simulink model "dcmotorsimexp"  (Simulink 5.0)
settings: Solver=ode45  SolverMode=SingleTasking  StartTime=0.0  StopTime=Tstop  RelTol=1e-3
values from neighbouring files (symbols this model uses):
  A = [-.0151 -60.5651 0 -32.174 ... (first row only)    [afti16.m]    (also in bmdp02.m = [0.7326   -0.0861; example4.m = [1 -1 0; regulator.m = [0 0; sphericle.m = [0 0 1 0;0 0 0 1 ;-66.2175 66.2175 -0.15 0 ;0 0 0 0])
  B = [-2.516 -13.136 ... (first row only)    [afti16.m]    (also in bmdp02.m = [0.0609;0.0064]; example4.m = [-1 1; regulator.m = [1;0]; sphericle.m = [0 0 0 1]')
  C = [0 1 0 0 ... (first row only)    [afti16.m]    (also in bmdp02.m = lincon(model,'reg',cost,interval,limits); example4.m = lincon(model,'reg',cost,interval,limits); mimo.m = lincon(model,'track',cost,interval,limits); regsiso.m = model.C)
  Cmotorexp = expcon(Cmotor,range,options)    [dcmotor.m]
  D = [0 0 ... (first row only)    [afti16.m]    (also in bmdp02.m = zeros(size(B)); example4.m = zeros(2,2); regulator.m = 0; sphericle.m = 0)
  Vmax = tauam*pi*dshaft^3/16    (= 78.5398163397)    [dcmotor.m]
  Vmin = -Vmax    (= -78.5398163397)    [dcmotor.m]
  x0 = zeros(4,1)    [afti16.m]    (also in bmdp02.m = [1 1]'; dcmotor.m; doubleint.m = [10,-.3]'; doubleintexp.m = [10,-.3]')
libraries: hyblib x1
settings Model: LastModifiedBy=Alberto Bemporad  ExtModeTrigMode=oneshot  ExtModeArmWhenConnect=off  LimitDataPoints=off  IntegerOverflowMsg=none  BooleanDataType=off

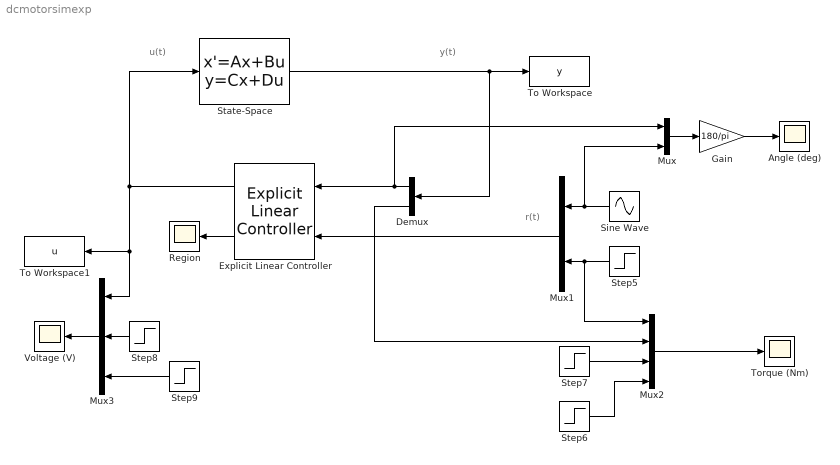
== system dcmotorsimexp ==
  note: u(t)
  note: y(t)
  note: r(t)
  Angle (deg) : Scope
      settings: TimeRange=20  YMin=-200  YMax=200  DataFormat=Structure
  Demux : Demux  Orientation=left  Outputs=2
  Explicit Linear Controller : hyblib/Explicit Linear Controller  Orientation=left  C=Cmotorexp  xhat0=[]  u1=[]  compile=on
  Gain : Gain  Gain=180/pi  SaturateOnIntegerOverflow=on
  Mux : Mux  Inputs=2
  Mux1 : Mux  Orientation=left  Inputs=2
  Mux2 : Mux
  Mux3 : Mux  Orientation=left  Inputs=3
  Region : Scope
      settings: TimeRange=20  YMin=0  YMax=80  DataFormat=Structure
  Sine Wave : Sin  Orientation=left  Amplitude=pi  Frequency=.4  SampleTime=0
  State-Space : StateSpace  A=A  B=B  C=C  D=D  X0=x0
  Step5 : Step  Orientation=left  Time=0  After=0  SampleTime=0
  Step6 : Step  Time=0  After=Vmin  SampleTime=0
  Step7 : Step  Time=0  After=Vmax  SampleTime=0
  Step8 : Step  Orientation=left  Time=0  After=220  SampleTime=0
  Step9 : Step  Orientation=left  Time=0  After=-220  SampleTime=0
  To Workspace : ToWorkspace  VariableName=y  SampleTime=-1  SaveFormat=Array
  To Workspace1 : ToWorkspace  VariableName=u  SampleTime=-1  SaveFormat=Array
  Torque (Nm) : Scope
      settings: TimeRange=20  YMin=-100  YMax=100  DataFormat=Structure
  Voltage (V) : Scope
      settings: TimeRange=20  YMin=-400  YMax=400  DataFormat=Structure
  wires:
  Mux/1 -> Gain/1
  Gain/1 -> Angle (deg)/1
  Mux2/1 -> Torque (Nm)/1
  Step5/1 -> Mux1/2, Mux2/1
  Mux1/1 -> Explicit Linear Controller/2
  Sine Wave/1 -> Mux1/1, Mux/2
  Step7/1 -> Mux2/3
  Step6/1 -> Mux2/4
  Mux3/1 -> Voltage (V)/1
  Step8/1 -> Mux3/2
  Step9/1 -> Mux3/3
  Explicit Linear Controller/1 -> To Workspace1/1, Mux3/1, State-Space/1
  State-Space/1 -> To Workspace/1, Demux/1
  Demux/1 -> Mux/1, Explicit Linear Controller/1
  Demux/2 -> Mux2/2
  Explicit Linear Controller/2 -> Region/1
